simulink model "Continuous_System_2"  (R2023a)
settings: Solver=VariableStepAuto  StartTime=0.0  StopTime=10.0  RelTol=1e-3
undefined symbols (not defined in the file): C, L, R
settings Model: Creator=Aman  LastModifiedBy=Aman

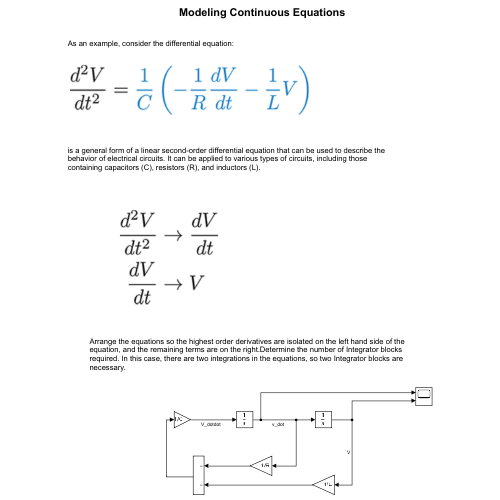
[thumbnail: Simulink's stored preview of the top-level diagram]
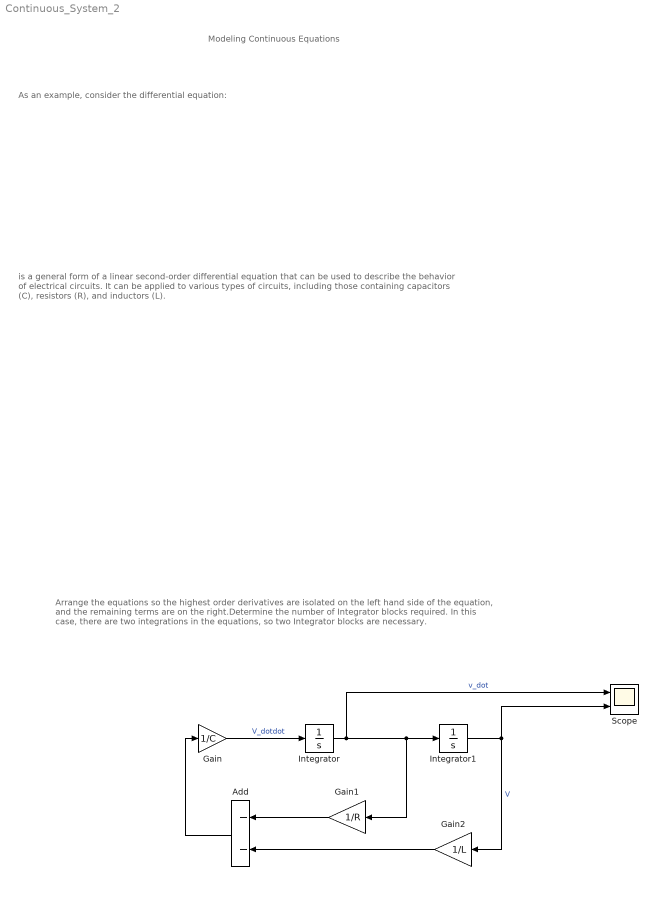
== system Continuous_System_2 ==
  note: is a general form of a linear second-order differential equation that can be used to describe the behavior of electrical circuits. It can be applied to various types of circuits, including those containing capacitors (C), resistors (R), and inductors (L).
  note: Arrange the equations so the highest order derivatives are isolated on the left hand side of the equation, and the remaining terms are on the right.Determine the number of Integrator blocks required. In this case, there are two integrations in the equations, so two Integrator blocks are necessary.
  note: As an example, consider the differential equation:
  note: Modeling Continuous Equations
  Add : Sum  Inputs=--
  Gain : Gain  Gain=1/C
  Gain1 : Gain  Gain=1/R
  Gain2 : Gain  Gain=1/L
  Integrator : Integrator
  Integrator1 : Integrator  InitialCondition=10
  Scope : Scope  NumInputPorts=2
  wires:
  Gain/1 -> Integrator/1  "V_dotdot"
  Integrator/1 -> Scope/1, Gain1/1, Integrator1/1  "v_dot"
  Gain1/1 -> Add/1
  Add/1 -> Gain/1
  Integrator1/1 -> Scope/2, Gain2/1  "V"
  Gain2/1 -> Add/2
